simulink model "model_2"  (R2023a)
settings: Solver=VariableStepAuto  StartTime=0.0  StopTime=0.1  RelTol=1e-3
settings Model: Creator=QUDUS  LastModifiedBy=QUDUS

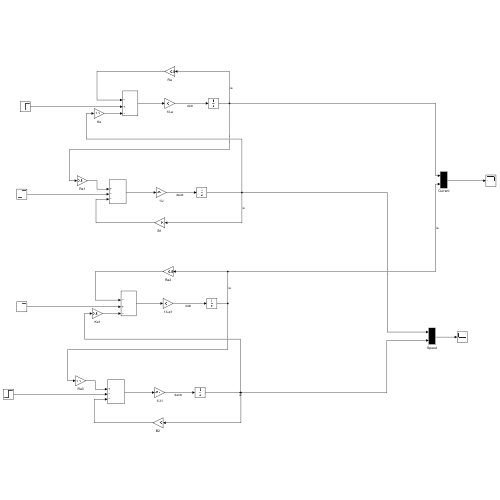
[thumbnail: Simulink's stored preview of the top-level diagram]
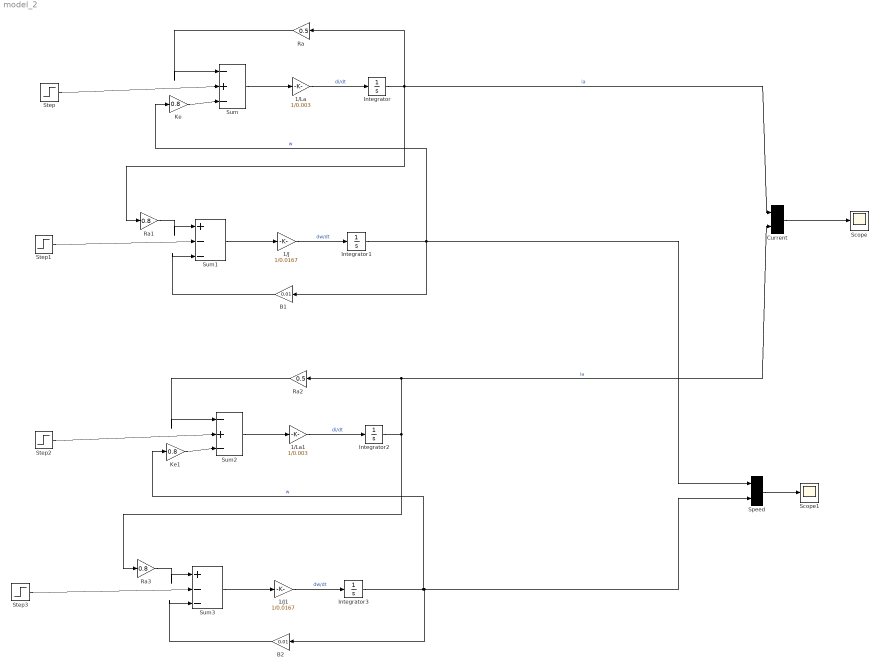
== system model_2 ==
  1/J : Gain  Gain=1/0.0167
  1/J1 : Gain  Gain=1/0.0167
  1/La : Gain  Gain=1/0.003
  1/La1 : Gain  Gain=1/0.003
  B1 : Gain  Gain=0.01
  B2 : Gain  Gain=0.01
  Current : Mux  Inputs=2
  Integrator{,1..3} (4 alike) : Integrator
  Ke : Gain  Gain=0.8
  Ke1 : Gain  Gain=0.8
  Ra : Gain  Gain=0.5
  Ra1 : Gain  Gain=0.8
  Ra2 : Gain  Gain=0.5
  Ra3 : Gain  Gain=0.8
  Scope : Scope
  Scope1 : Scope
  Speed : Mux  Inputs=2
  Step : Step  Time=0  After=220  SampleTime=0
  Step1 : Step  Time=0  After=0  SampleTime=0
  Step2 : Step  Time=0  After=220  SampleTime=0
  Step3 : Step  Time=0  After=100  SampleTime=0
  Sum : Sum  Inputs=|-+-
  Sum1 : Sum  Inputs=|+--
  Sum2 : Sum  Inputs=|-+-
  Sum3 : Sum  Inputs=|+--
  wires:
  Current/1 -> Scope/1
  Ke1/1 -> Sum2/3
  Sum2/1 -> 1/La1/1
  Step2/1 -> Sum2/2
  1/La1/1 -> Integrator2/1  "di/dt"
  Integrator2/1 -> Current/2, Ra2/1, Ra3/1  "ia"
  Sum3/1 -> 1/J1/1
  Ra3/1 -> Sum3/1
  B2/1 -> Sum3/3
  1/J1/1 -> Integrator3/1  "dw/dt"
  Speed/1 -> Scope1/1
  Step1/1 -> Sum1/2
  Step/1 -> Sum/2
  Ra/1 -> Sum/1
  1/La/1 -> Integrator/1  "di/dt"
  Sum/1 -> 1/La/1
  1/J/1 -> Integrator1/1  "dw/dt"
  Ke/1 -> Sum/3
  Step3/1 -> Sum3/2
  Ra1/1 -> Sum1/1
  B1/1 -> Sum1/3
  Integrator1/1 -> B1/1, Speed/1, Ke/1  "w"
  Sum1/1 -> 1/J/1
  Integrator/1 -> Ra1/1, Current/1, Ra/1  "ia"
  Integrator3/1 -> Ke1/1, Speed/2, B2/1  "w"
  Ra2/1 -> Sum2/1
